simulink model "penduleSimple_TP3_function"  (R2016a)
settings: Solver=FixedStepAuto  StartTime=t0  StopTime=tf  FixedStep=h  RelTol=1e-3
values from neighbouring files (symbols this model uses):
  alpha0 = 2*pi/10    (= 0.628318530718)    [init.m]
  g = -9.81    [init.m]    (also in init_TP1.m; init_TP2_controle.m; init_tp3.m; matrices_init_tp4_partie3_4.m = 9.81)
  h = (tf-t0)/N    [init.m]    (also in init_tp3.m)
  K = [100;10]    [init.m]    (also in init_TP2_controle.m = [20;10]; init_tp3.m = [20 10]; matrices_init_tp4_partie3_4.m = place(A,-B,V))
  l = 10    [init.m]    (also in init_TP1.m = 1; init_TP2_controle.m; init_tp3.m = 5)
  ue = 0    [init.m]    (also in init_TP2_controle.m; init_tp3.m)
  xe = [0;0]    [init.m]    (also in init_TP2_controle.m; init_tp3.m = [0 0])
undefined symbols (not defined in the file or in its folder): DiscIntNeverNeededParam
libraries: simulink x1
settings Model: Creator=fgaribal  LastModifiedBy=fgaribal

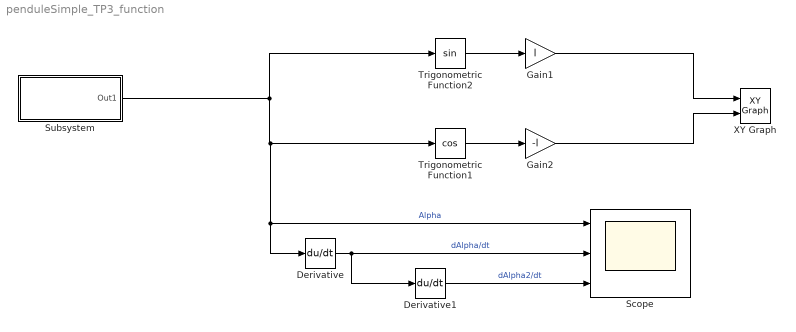
== system penduleSimple_TP3_function ==
  Derivative : Derivative
  Derivative1 : Derivative
  Gain1 : Gain  Gain=l
  Gain2 : Gain  Gain=-l
  Scope : Scope  NumInputPorts=3
  Subsystem : Subsystem
  Trigonometric Function1 : Trigonometry  Operator=cos
  Trigonometric Function2 : Trigonometry
  XY Graph : simulink/Sinks/XY Graph  xmin=-l  xmax=l  ymin=-l  ymax=l  st=-1
  wires:
  Trigonometric Function1/1 -> Gain2/1
  Trigonometric Function2/1 -> Gain1/1
  Gain2/1 -> XY Graph/2
  Gain1/1 -> XY Graph/1
  Subsystem/1(Out1) -> Derivative/1, Scope/1, Trigonometric Function1/1, Trigonometric Function2/1  "Alpha"
  Derivative/1 -> Derivative1/1, Scope/2  "dAlpha/dt"
  Derivative1/1 -> Scope/3  "dAlpha2/dt"

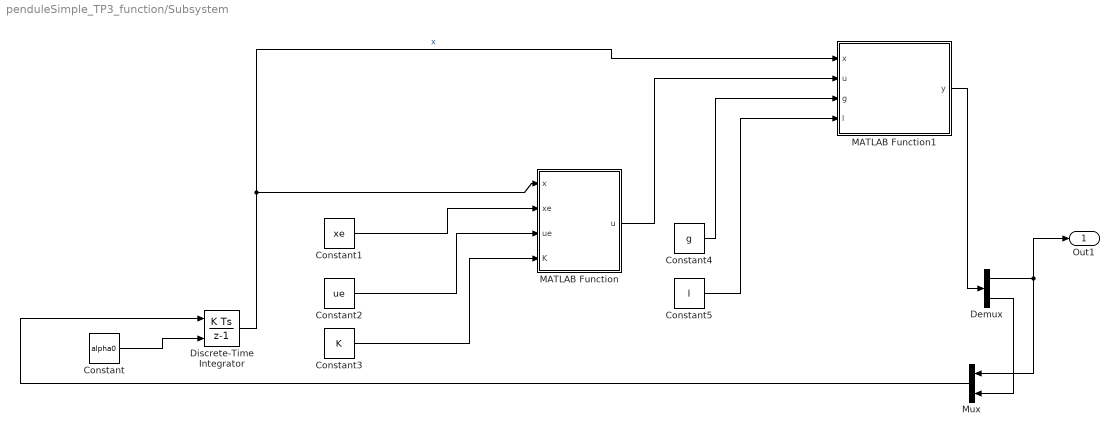
== system penduleSimple_TP3_function/Subsystem ==
  Constant : Constant  Value=alpha0
  Constant1 : Constant  Value=xe  VectorParams1D=off
  Constant2 : Constant  Value=ue
  Constant3 : Constant  Value=K  VectorParams1D=off
  Constant4 : Constant  Value=g
  Constant5 : Constant  Value=l
  Demux : Demux  Outputs=2
  Discrete-Time Integrator : DiscreteIntegrator  InitialConditionSource=external  InitialConditionSetting=State (most efficient)  SampleTime=h  ICPrevOutput=DiscIntNeverNeededParam  ICPrevScaledInput=DiscIntNeverNeededParam
  MATLAB Function : MATLAB Function  TreatAsAtomicUnit=on
  MATLAB Function1 : MATLAB Function  TreatAsAtomicUnit=on
  Mux : Mux  Inputs=2
  Out1 : Outport
  wires:
  Mux/1 -> Discrete-Time Integrator/1
  Demux/1 -> Out1/1, Mux/1
  MATLAB Function/1(u) -> MATLAB Function1/2(u)
  Discrete-Time Integrator/1 -> MATLAB Function/1(x), MATLAB Function1/1(x)  "x"
  MATLAB Function1/1(y) -> Demux/1
  Demux/2 -> Mux/2
  Constant1/1 -> MATLAB Function/2(xe)
  Constant2/1 -> MATLAB Function/3(ue)
  Constant3/1 -> MATLAB Function/4(K)
  Constant4/1 -> MATLAB Function1/3(g)
  Constant5/1 -> MATLAB Function1/4(l)
  Constant/1 -> Discrete-Time Integrator/2

== matlab function penduleSimple_TP3_function/Subsystem/MATLAB Function ==
  data: x input; u output; xe input; ue input; K input
function u = calcul_u(x, xe, ue, K)
    u = ue + K'*(x-xe);
end

== matlab function penduleSimple_TP3_function/Subsystem/MATLAB Function1 ==
  data: x input; u input; y output; g input; l input
function y = pendule_inverse(x,u,g,l)
    y = zeros(2,1);
    y(1)= x(2);
    y(2) = g/l*sin(x(1))-((u*cos(x(1)))/l);
end
